simulink model "PID_Controller"  (R2020b)
settings: Solver=VariableStepAuto  StartTime=0.0  StopTime=10.0  RelTol=1e-3
model workspace (MAT data in the model file):
  Kd = Simulink.Parameter
  Kd.Value = 484.0516
  Kd.DataType = 'auto'
  Kd.Dimensions = [1 1]
  Ki = Simulink.Parameter
  Ki.Value = 83.0917
  Ki.DataType = 'auto'
  Ki.Dimensions = [1 1]
  Kp = Simulink.Parameter
  Kp.Value = 495.0505
  Kp.DataType = 'auto'
  Kp.Dimensions = [1 1]
settings Model: ParameterArgumentNames=Kd,Ki,Kp  Creator=sayali  LastModifiedBy=sayali
settings DataIOCC: SaveOutput=off  SaveTime=off

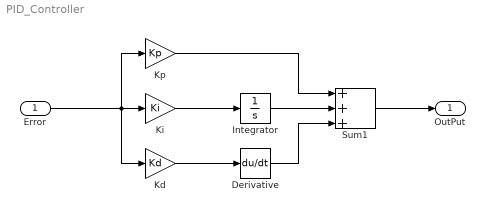
== system PID_Controller ==
  Error : Inport  OutDataTypeStr=double  PortDimensions=1  SampleTime=0
  Derivative : Derivative
  Integrator : Integrator
  Kd : Gain  Gain=Kd
  Ki : Gain  Gain=Ki
  Kp : Gain  Gain=Kp
  Sum1 : Sum  Inputs=+++
  OutPut : Outport  OutDataTypeStr=double  PortDimensions=1  SampleTime=0
  wires:
  Integrator/1 -> Sum1/2
  Kd/1 -> Derivative/1
  Derivative/1 -> Sum1/3
  Sum1/1 -> OutPut/1
  Ki/1 -> Integrator/1
  Kp/1 -> Sum1/1
  Error/1 -> Kp/1, Ki/1, Kd/1
